simulink model "v1"  (R2021b)
settings: Solver=VariableStepAuto  StartTime=0.0  StopTime=10  RelTol=1e-3
model workspace (MAT data in the model file):
  M_dry = 1
  g = 9.81
  m_fuel = 0.25
libraries: shared6dof x1, slpidlib x1
settings Model: Creator=josepfamador  LastModifiedBy=josepfamador

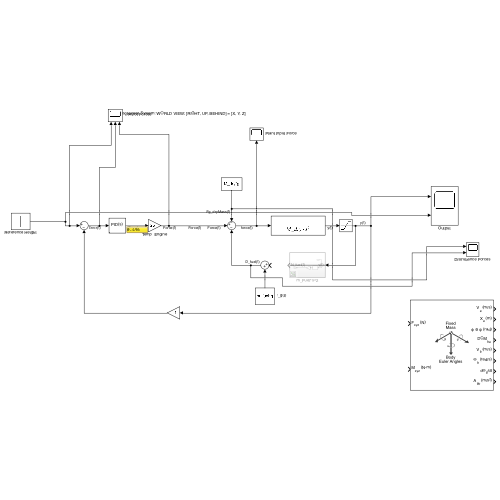
[thumbnail: Simulink's stored preview of the top-level diagram]
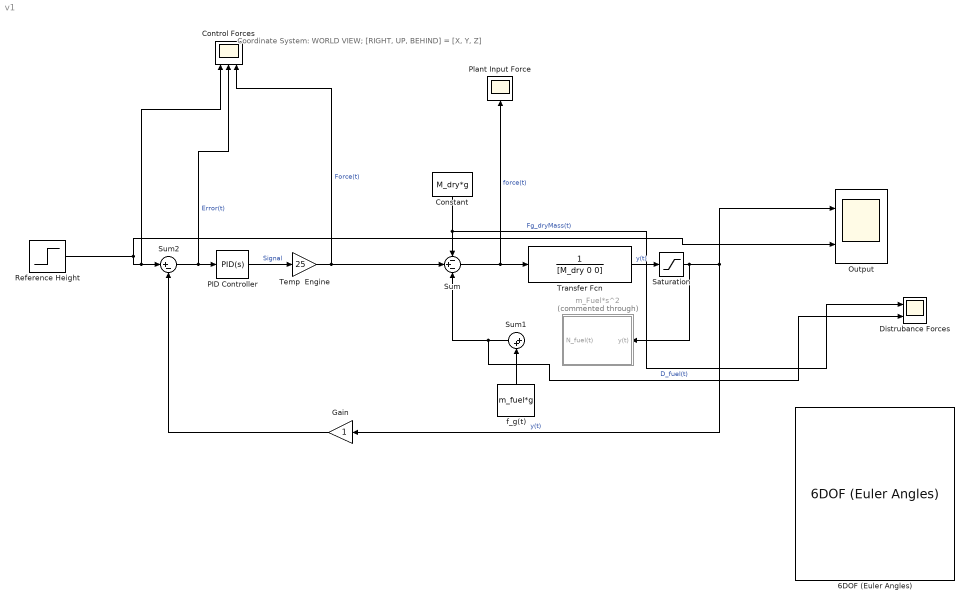
== system v1 ==
  note: Coordinate System: WORLD VIEW; [RIGHT, UP, BEHIND] = [X, Y, Z]
  6DOF (Euler Angles) : shared6dof/6DOF (Euler Angles)  units=Metric (MKS)  mtype=Fixed  rep=Euler Angles  xme_0=[0 0 0]  Vm_0=[0 0 0]  eul_0=[0 0 0]  pm_0=[0 0 0]  mass_0=1.0  mass_e=0.5  mass_f=2.0  inertia=eye(3)  inertia_e=eye(3)  inertia_f=2*eye(3)  k_quat=1.0  vre_flag=on  abi_flag=off  aMode=0  xme_statename=''  Vm_statename=''  eul_statename=''  quat_statename=''  pm_statename=''  mass_statename=''
      settings: SourceProductBaseCode=AE,PW,DR,MT,UV,VE
  Constant : Constant  Value=M_dry*g
  Control Forces : Scope  NumInputPorts=3
  Distrubance Forces : Scope  NumInputPorts=2
  Gain : Gain
  Output : Scope  NumInputPorts=2
  PID Controller : slpidlib/PID Controller  Controller=PID  Form=Parallel  TimeDomain=Continuous-time  UseExternalTs=off  SampleTime=-1  IntegratorMethod=Forward Euler  FilterMethod=Forward Euler  ControllerParametersSource=internal  P=0.372989398634807  I=0.10140866906395  D=0.315448885163463  UseFilter=on  N=100  TunerSelectOption=Transfer Function Based (PID Tuner App)  InitialConditionSource=internal  InitialConditionForIntegrator=1  InitialConditionForFilter=0  DifferentiatorICPrevScaledInput=0  ExternalReset=none  TrackingMode=off  Kt=1  LimitOutput=off  SatLimitsSource=internal  UpperSaturationLimit=30  LowerSaturationLimit=0  LinearizeAsGain=off  AntiWindupMode=none  Kb=1  POutMin=[]  POutMax=[]  IOutMin=[]  IOutMax=[]  DOutMin=[]  DOutMax=[]  NOutMin=[]  NOutMax=[]  SumOutMin=[]  SumOutMax=[]  SaturationOutMin=[]  SaturationOutMax=[]  PParamMin=[]  PParamMax=[]  IParamMin=[]  IParamMax=[]  DParamMin=[]  DParamMax=[]  NParamMin=[]  NParamMax=[]  KbParamMin=[]  KbParamMax=[]  KtParamMin=[]  KtParamMax=[]  KbOutMin=[]  KbOutMax=[]  KtOutMin=[]  KtOutMax=[]  IntegratorOutMin=[]  IntegratorOutMax=[]  FilterOutMin=[]  FilterOutMax=[]  SumI1OutMin=[]  SumI1OutMax=[]  SumI2OutMin=[]  SumI2OutMax=[]  SumI3OutMin=[]  SumI3OutMax=[]  SumI4OutMin=[]  SumI4OutMax=[]  SumDOutMin=[]  SumDOutMax=[]  DifferentiatorOutMin=[]  DifferentiatorOutMax=[]  FilterDiffOutCoefMin=[]  FilterDiffOutCoefMax=[]  ReciprocalOutMin=[]  ReciprocalOutMax=[]  SumDenOutMin=[]  SumDenOutMax=[]  SumNumOutMin=[]  SumNumOutMax=[]  DivideOutMin=[]  DivideOutMax=[]  UdiffTsProdOutMin=[]  UdiffTsProdOutMax=[]  NTsProdOutMin=[]  NTsProdOutMax=[]  UintegralTsProdOutMin=[]  UintegralTsProdOutMax=[]  UngainTsProdOutMin=[]  UngainTsProdOutMax=[]  IntegratorContinuousStateAttributes=''  IntegratorStateMustResolveToSignalObject=off  IntegratorRTWStateStorageClass=Auto  FilterContinuousStateAttributes=''  FilterStateMustResolveToSignalObject=off  FilterRTWStateStorageClass=Auto  ParallelPVariant=InternalParameters  IdealPVariant=Disabled  IVariant=InternalParameters  DVariant=InternalParameters  IntegratorVariant=Continuous  SatVariant=Disabled  AWVariant=Passthrough  PCopyVariant=Disabled  TRVariant=Disabled  FdbkBlocksVariant=Forward  IdealPFdbkVariant=Disabled  SatFdbkVariant=Disabled  DerivativeFilterVariant=ContFilter  NVariant=InternalParameters  NCopyVariant=Disabled  FilterICVariant=InternalICsFilter  IntegratorICVariant=InternalICs  ExternalResetVariant=Disabled  TRSumVariant=Passthrough  SumFdbkVariant=Disabled  SumVariant=Sum_PID  TsampFilterVariant=InternalTs  TsampNgainVariant=Passthrough  TsampIntegralVariant=Passthrough  ExternalSaturationOutDataTypeStr=Inherit: Same as second input
  Plant Input Force : Scope
  Reference Height : Step  SampleTime=0
  Saturation : Saturate  UpperLimit=inf  LowerLimit=0
  Sum : Sum  Inputs=-+-
  Sum1 : Sum  Inputs=|++
  Sum2 : Sum  Inputs=|+-
  Temp  Engine : Gain  Gain=25
  Transfer Fcn : TransferFcn  Denominator=[M_dry 0 0]  ContinuousStateAttributes="\"\""
  f_g(t) : Constant  Value=m_fuel*g
  m_Fuel*s^2 : Subsystem  Commented=through
  wires:
  PID Controller/1 -> Temp  Engine/1  "Signal"
  Sum/1 -> Transfer Fcn/1, Plant Input Force/1  "force(t)"
  Transfer Fcn/1 -> Saturation/1  "y(t)"
  Saturation/1 -> Output/1, Gain/1, m_Fuel*s^2/1(y(t))  "y(t)"
  f_g(t)/1 -> Sum1/2
  Sum1/1 -> Distrubance Forces/2, Sum/3  "D_fuel(t)"
  Constant/1 -> Distrubance Forces/1, Sum/1  "Fg_dryMass(t)"
  Reference Height/1 -> Sum2/1, Control Forces/1, Output/2
  Sum2/1 -> Control Forces/2, PID Controller/1  "Error(t)"
  Temp  Engine/1 -> Sum/2, Control Forces/3  "Force(t)"
  Gain/1 -> Sum2/2

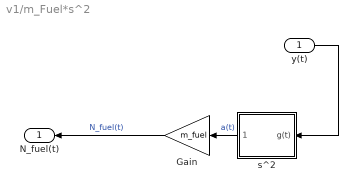
== system v1/m_Fuel*s^2 ==
  y(t) : Inport
  Gain : Gain  Gain=m_fuel
  s^2 : Subsystem
  N_fuel(t) : Outport
  wires:
  Gain/1 -> N_fuel(t)/1  "N_fuel(t)"
  y(t)/1 -> s^2/1(g(t))
  s^2/1(g2dot(t)) -> Gain/1  "a(t)"

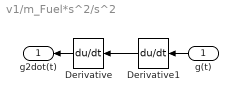
== system v1/m_Fuel*s^2/s^2 ==
  g(t) : Inport
  Derivative : Derivative
  Derivative1 : Derivative
  g2dot(t) : Outport
  wires:
  g(t)/1 -> Derivative1/1
  Derivative/1 -> g2dot(t)/1
  Derivative1/1 -> Derivative/1
